simulink model "Lab_4_2"  (R2021b)
settings: Solver=VariableStepAuto  StartTime=0.0  StopTime=10  RelTol=1e-3
libraries: spsRMSLib x6, spsPiSectionLineLib x3, spsPower3phInstantaneousLib x2, spsThreePhaseVIMeasurementLib x2, spsThreePhaseParallelRLCLoadLib x2, spsVoltageMeasurementLib x2, spsThreePhaseSourceLib x1, spspowerguiLib x1
settings Model: Creator=Lenovo  LastModifiedBy=coolk

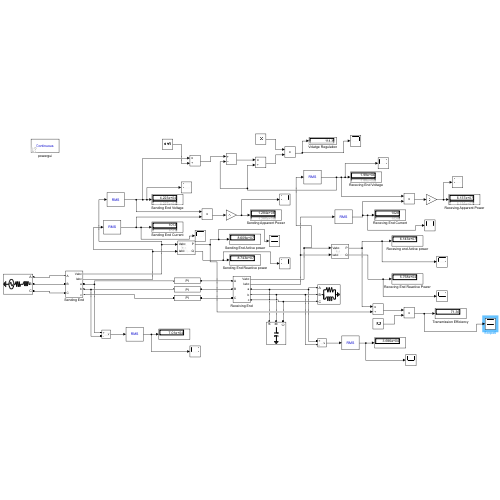
[thumbnail: Simulink's stored preview of the top-level diagram]
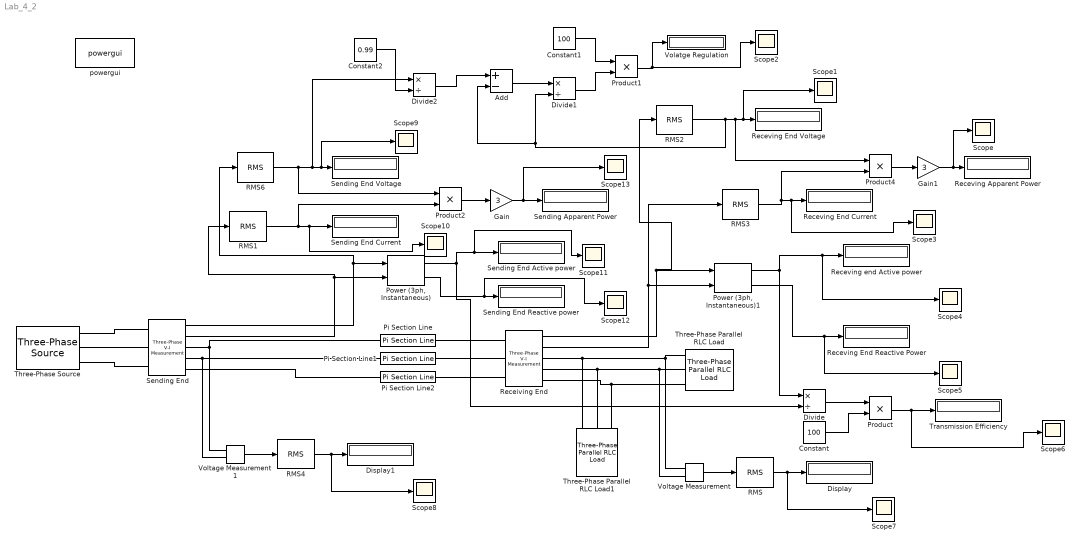
== system Lab_4_2 ==
  Add : Sum  Inputs=+-
  Constant : Constant  Value=100
  Constant1 : Constant  Value=100
  Constant2 : Constant  Value=0.99
  Display : Display
  Display1 : Display
  Divide : Product  Inputs=*/
  Divide1 : Product  Inputs=*/
  Divide2 : Product  Inputs=*/
  Gain : Gain  Gain=3
  Gain1 : Gain  Gain=3
  Pi Section Line : spsPiSectionLineLib/Pi Section Line  LConnTagsString=1  RConnTagsString=1  Phases=1  PiSections=1  Length=160  Frequency=50  Resistance=0.05501  Inductance=0.603e-3  Capacitance=0.01925e-6  Measurements=None  Measurements2=None
      settings: SourceProductBaseCode=PS
  Pi Section Line1 : spsPiSectionLineLib/Pi Section Line  LConnTagsString=1  RConnTagsString=1  Phases=1  PiSections=1  Length=160  Frequency=50  Resistance=0.05501  Inductance=0.603e-3  Capacitance=0.01925e-6  Measurements=None  Measurements2=None
      settings: SourceProductBaseCode=PS
  Pi Section Line2 : spsPiSectionLineLib/Pi Section Line  LConnTagsString=1  RConnTagsString=1  Phases=1  PiSections=1  Length=160  Frequency=50  Resistance=0.05501  Inductance=0.603e-3  Capacitance=0.01925e-6  Measurements=None  Measurements2=None
      settings: SourceProductBaseCode=PS
  "Power (3ph, Instantaneous)" : spsPower3phInstantaneousLib/Power (3ph, Instantaneous)
  "Power (3ph, Instantaneous)1" : spsPower3phInstantaneousLib/Power (3ph, Instantaneous)
  Product{,1..2,4} (4 alike) : Product
  RMS : spsRMSLib/RMS  TrueRMS=on  Freq=60  RMSInit=120  Ts=0
  RMS{1..3,6} (4 alike) : spsRMSLib/RMS  TrueRMS=on  Freq=50  RMSInit=0  Ts=0
  RMS4 : spsRMSLib/RMS  TrueRMS=on  Freq=60  RMSInit=120  Ts=0
  Receiving End : spsThreePhaseVIMeasurementLib/Three-Phase V-I Measurement  VoltageMeasurement=phase-to-ground  SetLabelV=off  LabelV=Vabc  Vpu=off  VpuLL=off  CurrentMeasurement=yes  SetLabelI=off  LabelI=Iabc  Ipu=off  Pbase=100e6  Vbase=500e3  OutputType=Complex  PhasorSimulation=off  PSBequivalent=0
  Receving Apparent Power : Display
  Receving End Current : Display
  Receving End Reactive Power : Display
  Receving End Voltage : Display
  Receving end Active power : Display
  Scope{,1..13} (14 alike) : Scope
  Sending Apparent Power : Display
  Sending End : spsThreePhaseVIMeasurementLib/Three-Phase V-I Measurement  VoltageMeasurement=phase-to-ground  SetLabelV=off  LabelV=Vabc  Vpu=off  VpuLL=off  CurrentMeasurement=yes  SetLabelI=off  LabelI=Iabc  Ipu=off  Pbase=100e6  Vbase=500e3  OutputType=Complex  PhasorSimulation=off  PSBequivalent=0
  Sending End Active power : Display
  Sending End Current : Display
  Sending End Reactive power : Display
  Sending End Voltage : Display
  Three-Phase Parallel RLC Load : spsThreePhaseParallelRLCLoadLib/Three-Phase Parallel RLC Load  LConnTagsString=A|B|C  Configuration=Y (grounded)  NominalVoltage=132e3  Vabc=[1e3 1e3 1e3]  Vabcp=[1e3 1e3 1e3]  NominalFrequency=50  UnbalancedPower=off  ActivePower=45e6*20  InductivePower=33.75e6  CapacitivePower=0  Pabc=[10e3 9e3 11e3]  QLabc=[100 90 110]  QCabc=[100 90 110]  Pabcp=[10e3 9e3 11e3]  QLabcp=[100 90 110]  QCabcp=[100 90 110]  Measurements=None  LoadType=constant Z
  Three-Phase Parallel RLC Load1 : spsThreePhaseParallelRLCLoadLib/Three-Phase Parallel RLC Load  LConnTagsString=A|B|C  Configuration=Y (grounded)  NominalVoltage=132e3  Vabc=[1e3 1e3 1e3]  Vabcp=[1e3 1e3 1e3]  NominalFrequency=50  UnbalancedPower=off  ActivePower=0  InductivePower=0  CapacitivePower=33.75e6  Pabc=[10e3 9e3 11e3]  QLabc=[100 90 110]  QCabc=[100 90 110]  Pabcp=[10e3 9e3 11e3]  QLabcp=[100 90 110]  QCabcp=[100 90 110]  Measurements=None  LoadType=constant Z
  Three-Phase Source : spsThreePhaseSourceLib/Three-Phase Source  InternalConnection=Yg  VoltagePhases=off  Voltage=80980  PhaseAngle=3.52  Voltage_phases=[25e3 25e3 25e3]/sqrt(3)  PhaseAngles_phases=[0 -120 +120]  Frequency=50  NonIdealSource=on  SpecifyImpedance=off  Resistance=0.8929  Inductance=16.58e-3  ShortCircuitLevel=100e6  BaseVoltage=25e3  XRratio=7  BusType=swing  Pref=10e3  Qref=0  Prefabc=[10e3, 10e3, 10e3]  Qrefabc=[0, 0, 0]  Qmin=-inf  Qmax=inf
  Transmission Efficiency : Display
  Volatge Regulation : Display
  Voltage Measurement : spsVoltageMeasurementLib/Voltage Measurement  PhasorSimulation=off  OutputType=Complex  PSBequivalent=0
  Voltage Measurement1 : spsVoltageMeasurementLib/Voltage Measurement  PhasorSimulation=off  OutputType=Complex  PSBequivalent=0
  powergui : spspowerguiLib/powergui  Priority=1  SimulationMode=Continuous  SampleTime=50e-6  frequency=60  Iterations=50  frequencyindice=50  Pbase=100e6  ErrMax=1e-4  UnitsV=kV  UnitsW=MW  buscounter=0  FunctionMessages=off  echomessages=off  EnableUseOfTLC=off  CurrentSourceSwitches=off  DisableSnubberDevices=off  DisableRonSwitches=off  DisableVfSwitches=off  DisplayEquations=off  AutomaticDiscreteSolvers=off  SolverType=Tustin/Backward Euler (TBE)  Interpol=off  ExternalGateDelay=off  methode=off  Ts=100  x0status=blocks  SPID=on  SwTol=0  HookPort=off  NonlinearTolerance=1e-4  nMaxIteration=100  ContinueOnMaxIteration=off  RestoreLinks=warning  ResistiveCurrentMeasurement=off  Frange=[0:2:500]  Ylog=off  Xlog=on  ShowGrid=off  save=off  variable=ZData  structure=0  ZoomFFT=off  StartTime=0.0  cycles=1  DisplayStyle=1  fundamental=60  FreqAxis=off  MaxFrequency=1000  frequencyindicesteady=1  RmsSteady=1  display=off
  wires:
  Sending End/1 -> RMS6/1, "Power (3ph, Instantaneous)"/1
  Sending End/2 -> RMS1/1, "Power (3ph, Instantaneous)"/2
  RMS6/1 -> Product2/1, Divide2/1, Scope9/1, Sending End Voltage/1
  RMS1/1 -> Product2/2, Scope10/1, Sending End Current/1
  "Power (3ph, Instantaneous)"/1 -> Scope11/1, Sending End Active power/1, Divide/2
  "Power (3ph, Instantaneous)"/2 -> Scope12/1, Sending End Reactive power/1
  RMS2/1 -> Add/2, Divide1/2, Product4/1, Scope1/1, Receving End Voltage/1
  "Power (3ph, Instantaneous)1"/2 -> Scope5/1, Receving End Reactive Power/1
  "Power (3ph, Instantaneous)1"/1 -> Scope4/1, Receving end Active power/1, Divide/1
  RMS3/1 -> Product4/2, Scope3/1, Receving End Current/1
  Receiving End/1 -> RMS2/1, "Power (3ph, Instantaneous)1"/1
  Receiving End/2 -> RMS3/1, "Power (3ph, Instantaneous)1"/2
  Divide/1 -> Product/1
  Constant/1 -> Product/2
  Product/1 -> Scope6/1, Transmission Efficiency/1
  Product1/1 -> Scope2/1, Volatge Regulation/1
  Constant1/1 -> Product1/1
  Divide1/1 -> Product1/2
  Add/1 -> Divide1/1
  Divide2/1 -> Add/1
  Constant2/1 -> Divide2/2
  Product2/1 -> Gain/1
  Gain/1 -> Scope13/1, Sending Apparent Power/1
  Gain1/1 -> Scope/1, Receving Apparent Power/1
  Product4/1 -> Gain1/1
  Voltage Measurement/1 -> RMS/1
  RMS/1 -> Scope7/1, Display/1
  Voltage Measurement1/1 -> RMS4/1
  RMS4/1 -> Scope8/1, Display1/1
  connections:
  Three-Phase Source/RConn1 -- Sending End/LConn1
  Three-Phase Source/RConn2 -- Sending End/LConn2
  Three-Phase Source/RConn3 -- Sending End/LConn3
  Three-Phase Parallel RLC Load/LConn2 -- Voltage Measurement/LConn2 -- Three-Phase Parallel RLC Load1/LConn2 -- Receiving End/RConn2
  Three-Phase Parallel RLC Load/LConn1 -- Voltage Measurement/LConn1 -- Three-Phase Parallel RLC Load1/LConn1 -- Receiving End/RConn1
  Three-Phase Parallel RLC Load/LConn3 -- Three-Phase Parallel RLC Load1/LConn3 -- Receiving End/RConn3
  Pi Section Line/RConn1 -- Receiving End/LConn1
  Pi Section Line1/RConn1 -- Receiving End/LConn2
  Pi Section Line2/RConn1 -- Receiving End/LConn3
  Sending End/RConn1 -- Pi Section Line/LConn1 -- Voltage Measurement1/LConn1
  Sending End/RConn2 -- Pi Section Line1/LConn1 -- Voltage Measurement1/LConn2
  Pi Section Line2/LConn1 -- Sending End/RConn3
